simulink model "guidance"  (Simulink 7.6)
settings: Solver=FixedStepDiscrete  StartTime=0.0  StopTime=Tfin  FixedStep=Ts  RelTol=1e-3
undefined symbols (not defined in the file or in its folder): heading_value, HOLD_HEADING
libraries: simulink x2
settings Model: Creator=Borja  LastModifiedBy=frafonal
settings OptimizationCC: InlineParams=on  OptimizeModelRefInitCode=on  LifeSpan=1
settings DebuggingCC: FcnCallInpInsideContextMsg=Enable All
settings RTWCC: SystemTargetFile=ert.tlc  GenCodeOnly=on  TemplateMakefile=ert_default_tmf  Description=Embedded Coder  ProcessScript=ert_make_rtw_hook
settings CodeAppCC: IgnoreCustomStorageClasses=off
settings ERTTargetCC: MultiwordLength=2048  GenerateSampleERTMain=on  SupportNonFinite=off  SupportComplex=off  InlinedParameterPlacement=NonHierarchical  ERTCustomFileTemplate=example_file_process.tlc  ConvertIfToSwitch=off

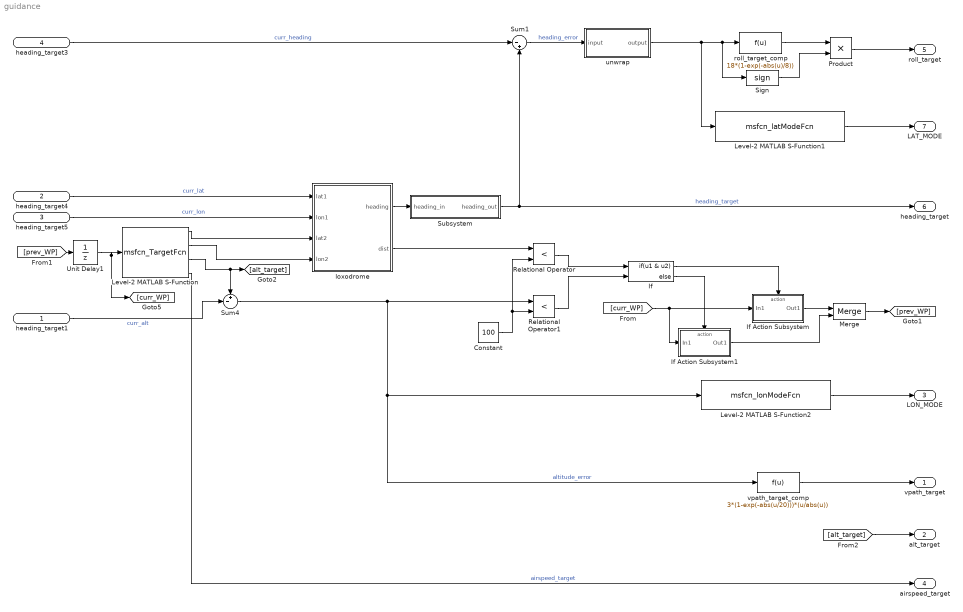
== system guidance ==
  heading_target1 : Inport
  heading_target4 : Inport  Port=2
  heading_target5 : Inport  Port=3
  heading_target3 : Inport  Port=4
  Constant : Constant  Value=100
  If : If  NumInputs=2  IfExpression=u1 & u2
  If Action Subsystem : Subsystem  TreatAsAtomicUnit=on
  If Action Subsystem1 : Subsystem  TreatAsAtomicUnit=on
  Level-2 MATLAB S-Function : M-S-Function  FunctionName=msfcn_TargetFcn  Parameters=wp,HOLD_ALT, HOLD_SPEED, alt_value, speed_value
      mask Display:
      | disp('Target')
      | port_label('input', 1, 'wp')
      | port_label('output', 1, 'lat')
      | port_label('output', 2, 'lon')
      | port_label('output', 3, 'alt')
      | port_label('output', 4, 'airspeed')
  Level-2 MATLAB S-Function1 : M-S-Function  FunctionName=msfcn_latModeFcn  Parameters=ROLL_CONTROL, HEADING_CONTROL
      mask Display:
      | disp('Lat Mode')
      | port_label('input', 1, 'heading error')
      | port_label('output', 1, 'mode')
  Level-2 MATLAB S-Function2 : M-S-Function  FunctionName=msfcn_lonModeFcn  Parameters=VPATH_CONTROL, ALT_CONTROL
      mask Display:
      | disp('Lat Mode')
      | port_label('input', 1, 'altitude error')
      | port_label('output', 1, 'mode')
  Merge : Merge
  Product : Product  RndMeth=Zero
  Relational Operator : RelationalOperator  Operator=<  OutDataTypeStr=boolean
  Relational Operator1 : RelationalOperator  Operator=<  OutDataTypeStr=boolean
  Sign : Signum
  Subsystem : Subsystem
  Sum1 : Sum  Inputs=|-+
  Sum4 : Sum  Inputs=+-|
  Unit Delay1 : UnitDelay  X0=1  SampleTime=-1
  loxodrome : Subsystem
  roll_target_comp : Fcn  Expr=18*(1-exp(-abs(u)/8))
  unwrap : Subsystem
  vpath_target_comp : Fcn  Expr=3*(1-exp(-abs(u/20)))*(u/abs(u))
  vpath_target : Outport
  alt_target : Outport  Port=2
  LON_MODE : Outport  Port=3
  airspeed_target : Outport  Port=4
  roll_target : Outport  Port=5
  heading_target : Outport  Port=6
  LAT_MODE : Outport  Port=7
  wires:
  heading_target3/1 -> Sum1/1  "curr_heading"
  Sum1/1 -> unwrap/1(input)  "heading_error"
  Level-2 MATLAB S-Function1/1 -> LAT_MODE/1
  unwrap/1(output) -> roll_target_comp/1, Sign/1, Level-2 MATLAB S-Function1/1
  Sum4/1 -> Relational Operator1/1, vpath_target_comp/1, Level-2 MATLAB S-Function2/1  "altitude_error"
  vpath_target_comp/1 -> vpath_target/1
  heading_target4/1 -> loxodrome/1(lat1)  "curr_lat"
  heading_target5/1 -> loxodrome/2(lon1)  "curr_lon"
  loxodrome/2(dist) -> Relational Operator/1
  Constant/1 -> Relational Operator/2, Relational Operator1/2
  Relational Operator/1 -> If/1
  Relational Operator1/1 -> If/2
  Unit Delay1/1 -> [curr_WP], Level-2 MATLAB S-Function/1
  heading_target1/1 -> Sum4/2  "curr_alt"
  If/2 -> If Action Subsystem1/Action
  If/1 -> If Action Subsystem/Action
  If Action Subsystem/1(Out1) -> Merge/1
  If Action Subsystem1/1(Out1) -> Merge/2
  Merge/1 -> [prev_WP]
  loxodrome/1(heading) -> Subsystem/1(heading_in)
  [curr_WP] -> If Action Subsystem/1(In1), If Action Subsystem1/1(In1)
  [prev_WP] -> Unit Delay1/1
  roll_target_comp/1 -> Product/1
  Product/1 -> roll_target/1
  Sign/1 -> Product/2
  [alt_target] -> alt_target/1
  Level-2 MATLAB S-Function2/1 -> LON_MODE/1
  Level-2 MATLAB S-Function/4 -> airspeed_target/1  "airspeed_target"
  Subsystem/1(heading_out) -> Sum1/2, heading_target/1  "heading_target"
  Level-2 MATLAB S-Function/1 -> loxodrome/3(lat2)
  Level-2 MATLAB S-Function/2 -> loxodrome/4(lon2)
  Level-2 MATLAB S-Function/3 -> [alt_target], Sum4/1

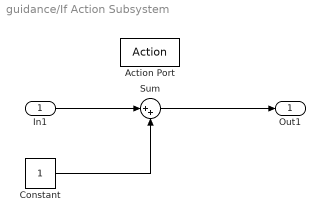
== system guidance/If Action Subsystem ==
  In1 : Inport
  Action Port : ActionPort  ActionType=then
  Constant : Constant
  Sum : Sum  Inputs=|++
  Out1 : Outport
  wires:
  Constant/1 -> Sum/2
  In1/1 -> Sum/1
  Sum/1 -> Out1/1

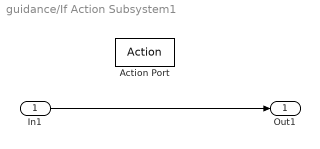
== system guidance/If Action Subsystem1 ==
  In1 : Inport
  Action Port : ActionPort  ActionType=else
  Out1 : Outport
  wires:
  In1/1 -> Out1/1

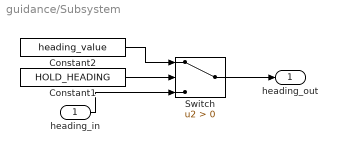
== system guidance/Subsystem ==
  heading_in : Inport
  Constant1 : Constant  Value=HOLD_HEADING
  Constant2 : Constant  Value=heading_value
  Switch : Switch  Criteria=u2 > Threshold
  heading_out : Outport
  wires:
  Constant1/1 -> Switch/2
  Constant2/1 -> Switch/1
  Switch/1 -> heading_out/1
  heading_in/1 -> Switch/3

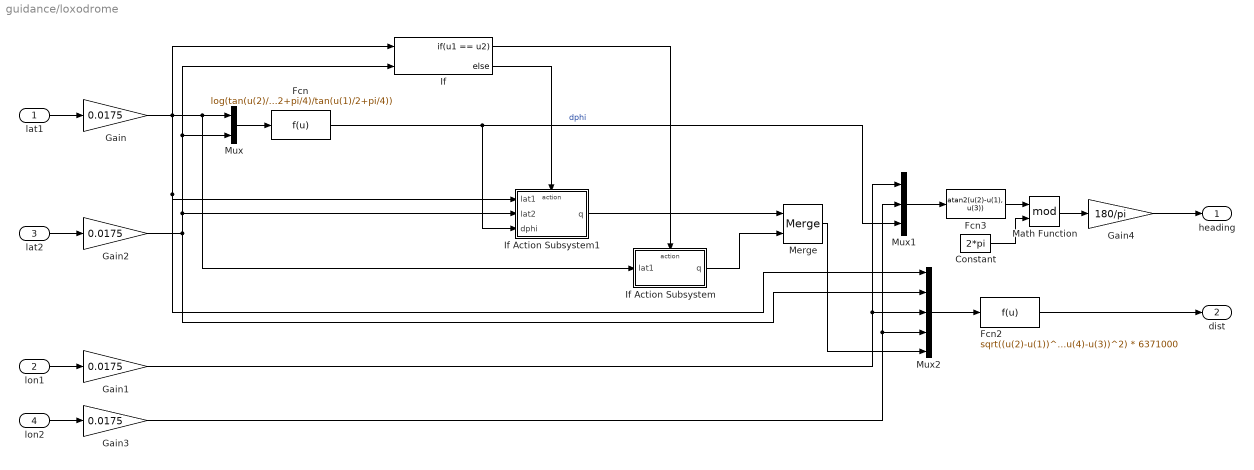
== system guidance/loxodrome ==
  lat1 : Inport
  lon1 : Inport  Port=2
  lat2 : Inport  Port=3
  lon2 : Inport  Port=4
  Constant : Constant  Value=2*pi
  Fcn : Fcn  Expr=log(tan(u(2)/2+pi/4)/tan(u(1)/2+pi/4))
  Fcn2 : Fcn  Expr=sqrt((u(2)-u(1))^2 + u(5)^2*(u(4)-u(3))^2) * 6371000
  Fcn3 : Fcn  Expr=atan2(u(2)-u(1), u(3))
  Gain{,1..3} (4 alike) : Gain  Gain=0.0175
  Gain4 : Gain  Gain=180/pi
  If : If  NumInputs=2  IfExpression=u1 == u2
  If Action Subsystem : Subsystem  TreatAsAtomicUnit=on
  If Action Subsystem1 : Subsystem  TreatAsAtomicUnit=on
  Math Function : Math  Operator=mod  SaturateOnIntegerOverflow=on
  Merge : Merge
  Mux : Mux  Inputs=2
  Mux1 : Mux  Inputs=3
  Mux2 : Mux  Inputs=5
  heading : Outport
  dist : Outport  Port=2
  wires:
  lat1/1 -> Gain/1
  lon1/1 -> Gain1/1
  lat2/1 -> Gain2/1
  lon2/1 -> Gain3/1
  Gain2/1 -> Mux2/2, Mux/2, If/2, If Action Subsystem1/2(lat2)
  Gain/1 -> Mux/1, If Action Subsystem/1(lat1), Mux2/1, If Action Subsystem1/1(lat1), If/1
  Mux/1 -> Fcn/1
  If/2 -> If Action Subsystem1/Action
  If/1 -> If Action Subsystem/Action
  If Action Subsystem/1(q) -> Merge/2
  If Action Subsystem1/1(q) -> Merge/1
  Mux1/1 -> Fcn3/1
  Merge/1 -> Mux2/5
  Gain1/1 -> Mux1/1, Mux2/3
  Gain3/1 -> Mux1/2, Mux2/4
  Mux2/1 -> Fcn2/1
  Fcn2/1 -> dist/1
  Fcn/1 -> If Action Subsystem1/3(dphi), Mux1/3  "dphi"
  Fcn3/1 -> Math Function/1
  Math Function/1 -> Gain4/1
  Constant/1 -> Math Function/2
  Gain4/1 -> heading/1

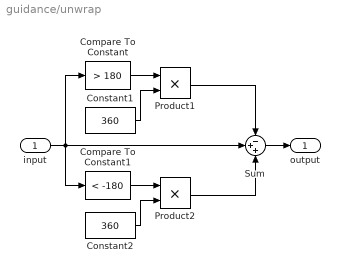
== system guidance/unwrap ==
  input : Inport
  Compare To Constant : simulink/Logic and Bit Operations/Compare To Constant  SystemSampleTime=-1  relop=>  const=180  LogicOutDataTypeMode=uint8
  Compare To Constant1 : simulink/Logic and Bit Operations/Compare To Constant  SystemSampleTime=-1  relop=<  const=-180  LogicOutDataTypeMode=uint8
  Constant1 : Constant  Value=360
  Constant2 : Constant  Value=360
  Product1 : Product  RndMeth=Zero
  Product2 : Product  RndMeth=Zero
  Sum : Sum  Inputs=-++
  output : Outport
  wires:
  Compare To Constant/1 -> Product1/1
  Constant1/1 -> Product1/2
  Compare To Constant1/1 -> Product2/1
  Constant2/1 -> Product2/2
  Product1/1 -> Sum/1
  Product2/1 -> Sum/3
  Sum/1 -> output/1
  input/1 -> Sum/2, Compare To Constant/1, Compare To Constant1/1

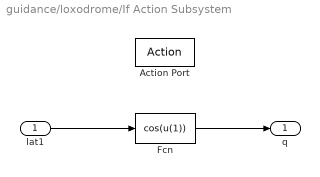
== system guidance/loxodrome/If Action Subsystem ==
  lat1 : Inport
  Action Port : ActionPort  ActionType=then
  Fcn : Fcn  Expr=cos(u(1))
  q : Outport
  wires:
  lat1/1 -> Fcn/1
  Fcn/1 -> q/1

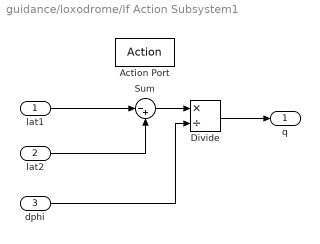
== system guidance/loxodrome/If Action Subsystem1 ==
  lat1 : Inport
  lat2 : Inport  Port=2
  dphi : Inport  Port=3
  Action Port : ActionPort  ActionType=else
  Divide : Product  Inputs=*/
  Sum : Sum  Inputs=|-+
  q : Outport
  wires:
  lat1/1 -> Sum/1
  lat2/1 -> Sum/2
  Sum/1 -> Divide/1
  dphi/1 -> Divide/2
  Divide/1 -> q/1
